simulink model "e5_Quadrotor_stable_nn"  (R2020a)
settings: Solver=FixedStepAuto  StartTime=0.0  StopTime=options.T_train  FixedStep=options.dt  RelTol=1e-6
undefined symbols (not defined in the file or in its folder): options, Quad
libraries: neural x123, simulink x3
(part 1 of 7)
settings Model: Creator=test  LastModifiedBy=kekatos
settings DataIOCC: LimitDataPoints=on  SaveFormat=Array  SignalLoggingSaveFormat=ModelDataLogs  ReturnWorkspaceOutputs=off
settings OptimizationCC: ExpressionDepthLimit=2147483647  LifeSpan=inf
settings DebuggingCC: UnderspecifiedInitializationDetection=Classic  MergeDetectMultiDrivingBlocksExec=none  SolverPrmCheckMsg=warning  FcnCallInpInsideContextMsg=warning  StateNameClashWarn=warning  SFUnexpectedBacktrackingDiag=warning  SFNoUnconditionalDefaultTransitionDiag=warning  SFExecutionAtInitializationDiag=none  ArithmeticOperatorsInVariantConditions=warning
settings HardwareCC: ProdBitPerPointer=32  ProdBitPerSizeT=32  ProdBitPerPtrDiffT=32  ProdLargestAtomicFloat=None  ProdIntDivRoundTo=Undefined  ProdEndianess=Unspecified  ProdWordSize=32  ProdHWDeviceType=32-bit Generic
settings ModelReferenceCC: PropagateSignalLabelsOutOfModel=off
settings SFSimCC: SimUseLocalCustomCode=off  CustomCodeUndefinedFunction=UseInterfaceOnly
settings RTWCC: RTWUseLocalCustomCode=off
settings CodeAppCC: StateflowObjectComments=on
settings GRTTargetCC: TargetLangStandard=C89/C90 (ANSI)  CombineOutputUpdateFcns=off  GRTInterface=on
settings ConfigComp: CovMetricSettings=dw  CovHtmlReporting=on  CovSaveCumulativeToWorkspaceVar=on  CovSaveSingleToWorkspaceVar=on

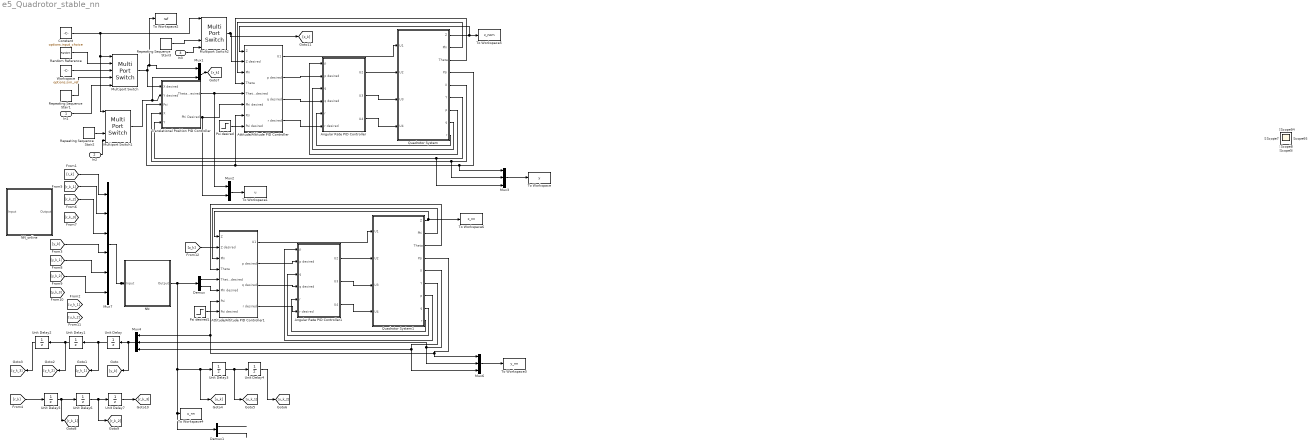
== system e5_Quadrotor_stable_nn ==
  In1 : Inport
  In2 : Inport  Port=2
  In3 : Inport  Port=3
  Angular Rate PID Controller : Subsystem
  Angular Rate PID Controller1 : Subsystem
  Attitude/Altitude PID Controller : Subsystem
  Attitude/Altitude PID Controller1 : Subsystem
  Constant : Constant  Value=options.input_choice
  Demux : Demux  Outputs=2
  Demux1 : Demux  Outputs=2
  Multiport Switch : MultiPortSwitch  Inputs=4
  Multiport Switch1 : MultiPortSwitch  Inputs=4
  Multiport Switch2 : MultiPortSwitch  Inputs=4
  Mux1 : Mux  Inputs=2
  Mux2 : Mux  Inputs=2
  Mux3 : Mux  Inputs=3
  Mux4 : Mux  Inputs=3
  Mux6 : Mux  Inputs=3
  Mux7 : Mux  Inputs=6
  NN : Subsystem
      mask help: Feed-Forward Neural Network
      mask Display: e = 0.06;c1 = [120 150 230]/255;c2 = ([120 150 230]+0)/383;c3 = ([120 150 230]+128)/383;patch([0 1 1 0],[0 0 1 1],c1);patch([0 1 1 1-e 1-e 0+e],[0 0 1 1-e 0+e 0+e],c2);patch([0 0 1 1-e 0+e 0+e],[0 1 1 1-e 1-e 0+e],c3);plot([0 1 1 0 0],[0 0 1 1 0]);fprintf('NNET');port_label('input',1,' Input');port_label('output',1,'Output ');
  NN_online : Subsystem
      mask help: Feed-Forward Neural Network
      mask Display: e = 0.06;c1 = [120 150 230]/255;c2 = ([120 150 230]+0)/383;c3 = ([120 150 230]+128)/383;patch([0 1 1 0],[0 0 1 1],c1);patch([0 1 1 1-e 1-e 0+e],[0 0 1 1-e 0+e 0+e],c2);patch([0 0 1 1-e 0+e 0+e],[0 1 1 1-e 1-e 0+e],c3);plot([0 1 1 0 0],[0 0 1 1 0]);fprintf('NNET');port_label('input',1,' Input');port_label('output',1,'Output ');
  Psi desired : Step  After=0  SampleTime=0
  Psi desired1 : Step  After=0  SampleTime=0
  Quadrotor System : Subsystem
  Quadrotor System1 : Subsystem
  Random Reference : UniformRandomNumber  Minimum=options.ref_min  Maximum=options.ref_max  Seed=randi(2^32,[1 ])  SampleTime=options.ref_Ts
  Repeating Sequence Stair1 : simulink/Sources/Repeating Sequence Stair  OutValues=options.sim_cov  tsamp=options.ref_Ts  OutMin=[]  OutMax=[]  OutDataTypeStr=double  OutputDataTypeScalingMode=double  OutDataType=fixdt(0,8)  ConRadixGroup=Best Precision: Vector-wise  OutScaling=2^-12
  Repeating Sequence Stair2 : simulink/Sources/Repeating Sequence Stair  OutValues=[0.0286;0.0154]  tsamp=options.ref_Ts  OutMin=[]  OutMax=[]  OutDataTypeStr=double  OutputDataTypeScalingMode=double  OutDataType=fixdt(0,8)  ConRadixGroup=Best Precision: Vector-wise  OutScaling=2^-12
  Repeating Sequence Stair3 : simulink/Sources/Repeating Sequence Stair  OutValues=[0.0286;0.0154]  tsamp=options.ref_Ts  OutMin=[]  OutMax=[]  OutDataTypeStr=double  OutputDataTypeScalingMode=double  OutDataType=fixdt(0,8)  ConRadixGroup=Best Precision: Vector-wise  OutScaling=2^-12
  To Workspace : ToWorkspace  VariableName=y  SaveFormat=Structure With Time  SampleTime=0.01
  To Workspace1 : ToWorkspace  VariableName=u  SaveFormat=Structure With Time  SampleTime=0.01
  To Workspace2 : ToWorkspace  VariableName=ref  SaveFormat=Structure With Time  SampleTime=0.01
  To Workspace3 : ToWorkspace  VariableName=y_nn  SaveFormat=Structure With Time  SampleTime=0.01
  To Workspace4 : ToWorkspace  VariableName=u_nn  SaveFormat=Structure With Time  SampleTime=0.01
  To Workspace5 : ToWorkspace  VariableName=z_nom  SaveFormat=Structure With Time  SampleTime=0.01
  To Workspace6 : ToWorkspace  VariableName=z_nn  SaveFormat=Structure With Time  SampleTime=0.01
  Translational Position PID Controller : Subsystem
  Unit Delay{,1..7} (8 alike) : UnitDelay  SampleTime=-1  HasFrameUpgradeWarning=on
  Workspace : Constant  Value=options.sim_ref
  Scope{,1..16} (17 alike) : Scope
  wires:
  Quadrotor System/2(Phi) -> Attitude/Altitude PID Controller/3(Phi)
  Quadrotor System/3(Theta) -> Attitude/Altitude PID Controller/4(Theta)
  Quadrotor System/4(Psi) -> Mux3/1, Translational Position PID Controller/3(Psi), Attitude/Altitude PID Controller/7(Psi)
  Quadrotor System/5(X) -> Mux3/2, Translational Position PID Controller/4(X)
  Quadrotor System/6(Y) -> Mux3/3, Translational Position PID Controller/5(Y)
  Quadrotor System/1(Z) -> To Workspace5/1, Attitude/Altitude PID Controller/1(Z)
  Psi desired/1 -> Attitude/Altitude PID Controller/8(Psi desired)
  Attitude/Altitude PID Controller/1(U1) -> Quadrotor System/1(U1)
  Translational Position PID Controller/1(Theta Desired) -> Mux2/1, Attitude/Altitude PID Controller/5(Theta desired)
  Translational Position PID Controller/2(Phi Desired) -> Attitude/Altitude PID Controller/6(Phi desired), Mux2/2
  Attitude/Altitude PID Controller/2(p desired) -> Angular Rate PID Controller/2(p desired)
  Attitude/Altitude PID Controller/3(q desired) -> Angular Rate PID Controller/4(q desired)
  Attitude/Altitude PID Controller/4(r desired) -> Angular Rate PID Controller/6(r desired)
  Quadrotor System/9(r) -> Angular Rate PID Controller/5(r)
  Quadrotor System/8(q) -> Angular Rate PID Controller/3(q)
  Quadrotor System/7(p) -> Angular Rate PID Controller/1(p)
  Angular Rate PID Controller/3(U4) -> Quadrotor System/4(U4)
  Angular Rate PID Controller/2(U3) -> Quadrotor System/3(U3)
  Angular Rate PID Controller/1(U2) -> Quadrotor System/2(U2)
  Mux2/1 -> To Workspace1/1
  Mux3/1 -> To Workspace/1
  In1/1 -> Multiport Switch/5
  Workspace/1 -> Multiport Switch/3
  Random Reference/1 -> Multiport Switch/2
  Repeating Sequence Stair1/1 -> Multiport Switch/4
  Constant/1 -> Multiport Switch2/1, Multiport Switch1/1, Multiport Switch/1
  Attitude/Altitude PID Controller1/2(p desired) -> Angular Rate PID Controller1/2(p desired)
  Attitude/Altitude PID Controller1/1(U1) -> Quadrotor System1/1(U1)
  Psi desired1/1 -> Attitude/Altitude PID Controller1/8(Psi desired)
  Quadrotor System1/9(r) -> Angular Rate PID Controller1/5(r)
  Quadrotor System1/6(Y) -> Mux4/3, Mux6/3
  Angular Rate PID Controller1/2(U3) -> Quadrotor System1/3(U3)
  Demux/1 -> Attitude/Altitude PID Controller1/5(Theta desired)
  Attitude/Altitude PID Controller1/3(q desired) -> Angular Rate PID Controller1/4(q desired)
  Quadrotor System1/7(p) -> Angular Rate PID Controller1/1(p)
  Quadrotor System1/2(Phi) -> Attitude/Altitude PID Controller1/3(Phi)
  Quadrotor System1/4(Psi) -> Mux6/1, Mux4/1, Attitude/Altitude PID Controller1/7(Psi)
  Demux/2 -> Attitude/Altitude PID Controller1/6(Phi desired)
  Quadrotor System1/3(Theta) -> Attitude/Altitude PID Controller1/4(Theta)
  Angular Rate PID Controller1/1(U2) -> Quadrotor System1/2(U2)
  Quadrotor System1/5(X) -> Mux4/2, Mux6/2
  Angular Rate PID Controller1/3(U4) -> Quadrotor System1/4(U4)
  Quadrotor System1/1(Z) -> Attitude/Altitude PID Controller1/1(Z), To Workspace6/1
  Attitude/Altitude PID Controller1/4(r desired) -> Angular Rate PID Controller1/6(r desired)
  NN/1(Output) -> [u_k], Unit Delay3/1, Demux1/1, To Workspace4/1, Demux/1
  Mux6/1 -> To Workspace3/1
  Quadrotor System1/8(q) -> Angular Rate PID Controller1/3(q)
  Multiport Switch/1 -> Translational Position PID Controller/1(X desired), Mux1/1, To Workspace2/1
  Mux4/1 -> Unit Delay/1, [y_k]
  [r_k] -> Mux7/1
  Mux1/1 -> [r_k]
  Unit Delay/1 -> Unit Delay1/1, [y_k_1]
  Unit Delay1/1 -> Unit Delay2/1, [y_k_2]
  Unit Delay2/1 -> [y_k_3]
  Unit Delay3/1 -> [u_k_1], Unit Delay4/1
  Unit Delay4/1 -> [u_k_2]
  [r_k] -> Unit Delay5/1
  Unit Delay5/1 -> [r_k_1], Unit Delay6/1
  Unit Delay6/1 -> [r_k_2], Unit Delay7/1
  Unit Delay7/1 -> [r_k_3]
  [r_k_1] -> Mux7/2
  [r_k_2] -> Mux7/3
  [y_k] -> Mux7/4
  [y_k_1] -> Mux7/5
  Demux1/1 -> ?
  Demux1/2 -> ?
  Multiport Switch1/1 -> Mux1/2, Translational Position PID Controller/2(Y desired)
  In2/1 -> Multiport Switch1/5
  Repeating Sequence Stair2/1 -> Multiport Switch1/4
  Repeating Sequence Stair3/1 -> Multiport Switch2/4
  In3/1 -> Multiport Switch2/5
  Multiport Switch2/1 -> [z_k], Attitude/Altitude PID Controller/2(Z desired)
  [y_k_2] -> Mux7/6
  [z_k] -> Attitude/Altitude PID Controller1/2(Z desired)
  Mux7/1 -> NN/1(Input)

== system e5_Quadrotor_stable_nn/Angular Rate PID Controller ==
  p : Inport
  p desired : Inport  Port=2
  q : Inport  Port=3
  q desired : Inport  Port=4
  r : Inport  Port=5
  r desired : Inport  Port=6
  p PID : Subsystem
  q PID : Subsystem
  r PID : Subsystem
  U2 : Outport  VectorParamsAs1DForOutWhenUnconnected=off
  U3 : Outport  Port=2  VectorParamsAs1DForOutWhenUnconnected=off
  U4 : Outport  Port=3  VectorParamsAs1DForOutWhenUnconnected=off
  wires:
  p PID/1(U2) -> U2/1
  q PID/1(U3) -> U3/1
  r PID/1(U4) -> U4/1
  p/1 -> p PID/1(p)
  p desired/1 -> p PID/2(p desired)
  q/1 -> q PID/1(q)
  q desired/1 -> q PID/2(q desired)
  r/1 -> r PID/1(r)
  r desired/1 -> r PID/2(r desired)

== system e5_Quadrotor_stable_nn/Angular Rate PID Controller1 ==
  p : Inport
  p desired : Inport  Port=2
  q : Inport  Port=3
  q desired : Inport  Port=4
  r : Inport  Port=5
  r desired : Inport  Port=6
  p PID : Subsystem
  q PID : Subsystem
  r PID : Subsystem
  U2 : Outport  VectorParamsAs1DForOutWhenUnconnected=off
  U3 : Outport  Port=2  VectorParamsAs1DForOutWhenUnconnected=off
  U4 : Outport  Port=3  VectorParamsAs1DForOutWhenUnconnected=off
  wires:
  p PID/1(U2) -> U2/1
  q PID/1(U3) -> U3/1
  r PID/1(U4) -> U4/1
  p/1 -> p PID/1(p)
  p desired/1 -> p PID/2(p desired)
  q/1 -> q PID/1(q)
  q desired/1 -> q PID/2(q desired)
  r/1 -> r PID/1(r)
  r desired/1 -> r PID/2(r desired)

== system e5_Quadrotor_stable_nn/Attitude//Altitude PID Controller ==
  Z : Inport
  Z desired : Inport  Port=2
  Phi : Inport  Port=3
  Theta : Inport  Port=4
  Theta desired : Inport  Port=5
  Phi desired : Inport  Port=6
  Psi : Inport  Port=7
  Psi desired : Inport  Port=8
  Phi PID : Subsystem
  Psi PID : Subsystem
  Theta PID : Subsystem
  Z PID : Subsystem
  U1 : Outport  VectorParamsAs1DForOutWhenUnconnected=off
  p desired : Outport  Port=2  VectorParamsAs1DForOutWhenUnconnected=off
  q desired : Outport  Port=3  VectorParamsAs1DForOutWhenUnconnected=off
  r desired : Outport  Port=4  VectorParamsAs1DForOutWhenUnconnected=off
  wires:
  Z PID/1(U1) -> U1/1
  Z desired/1 -> Z PID/2(Z desired)
  Z/1 -> Z PID/1(Z)
  Phi desired/1 -> Phi PID/2(Phi desired)
  Phi/1 -> Phi PID/1(Phi), Z PID/3(Phi)
  Psi desired/1 -> Psi PID/2(Psi desired)
  Psi/1 -> Psi PID/1(Psi)
  Theta desired/1 -> Theta PID/2(Theta desired)
  Theta/1 -> Theta PID/1(Theta), Z PID/4(Theta)
  Phi PID/1(p desired) -> p desired/1
  Psi PID/1(r desired) -> r desired/1
  Theta PID/1(q desired) -> q desired/1

== system e5_Quadrotor_stable_nn/Attitude//Altitude PID Controller1 ==
  Z : Inport
  Z desired : Inport  Port=2
  Phi : Inport  Port=3
  Theta : Inport  Port=4
  Theta desired : Inport  Port=5
  Phi desired : Inport  Port=6
  Psi : Inport  Port=7
  Psi desired : Inport  Port=8
  Phi PID : Subsystem
  Psi PID : Subsystem
  Theta PID : Subsystem
  Z PID : Subsystem
  U1 : Outport  VectorParamsAs1DForOutWhenUnconnected=off
  p desired : Outport  Port=2  VectorParamsAs1DForOutWhenUnconnected=off
  q desired : Outport  Port=3  VectorParamsAs1DForOutWhenUnconnected=off
  r desired : Outport  Port=4  VectorParamsAs1DForOutWhenUnconnected=off
  wires:
  Z PID/1(U1) -> U1/1
  Z desired/1 -> Z PID/2(Z desired)
  Z/1 -> Z PID/1(Z)
  Phi desired/1 -> Phi PID/2(Phi desired)
  Phi/1 -> Phi PID/1(Phi), Z PID/3(Phi)
  Psi desired/1 -> Psi PID/2(Psi desired)
  Psi/1 -> Psi PID/1(Psi)
  Theta desired/1 -> Theta PID/2(Theta desired)
  Theta/1 -> Theta PID/1(Theta), Z PID/4(Theta)
  Phi PID/1(p desired) -> p desired/1
  Psi PID/1(r desired) -> r desired/1
  Theta PID/1(q desired) -> q desired/1

== system e5_Quadrotor_stable_nn/NN ==
  Input : Inport  PortDimensions=15
      mask Display: e = 0.06;c1 = [120 230 180]/255;c2 = ([120 230 180]+0)/(256+128);c3 = ([120 230 180]+128)/(256+128);patch([0 1 1 0],[0 0 1 1],c1);patch([0 1 1 1-e 1-e 0+e],[0 0 1 1-e 0+e 0+e],c2);patch([0 0 1 1-e 0+e 0+e],[0 1 1 1-e 1-e 0+e],c3);plot([0 1 1 0 0],[0 0 1 1 0]);
  Layer 1 : Subsystem
      mask Display: e = 0.06;c1 = [120 150 230]/255;c2 = ([120 150 230]+0)/383;c3 = ([120 150 230]+128)/383;patch([0 1 1 0],[0 0 1 1],c1);patch([0 1 1 1-e 1-e 0+e],[0 0 1 1-e 0+e 0+e],c2);patch([0 0 1 1-e 0+e 0+e],[0 1 1 1-e 1-e 0+e],c3);plot([0 1 1 0 0],[0 0 1 1 0]);
  Layer 2 : Subsystem
      mask Display: e = 0.06;c1 = [120 150 230]/255;c2 = ([120 150 230]+0)/383;c3 = ([120 150 230]+128)/383;patch([0 1 1 0],[0 0 1 1],c1);patch([0 1 1 1-e 1-e 0+e],[0 0 1 1-e 0+e 0+e],c2);patch([0 0 1 1-e 0+e 0+e],[0 1 1 1-e 1-e 0+e],c3);plot([0 1 1 0 0],[0 0 1 1 0]);
  Process Input 1 : Subsystem
      mask Display: e = 0.06;c1 = [120 150 230]/255;c2 = ([120 150 230]+0)/383;c3 = ([120 150 230]+128)/383;patch([0 1 1 0],[0 0 1 1],c1);patch([0 1 1 1-e 1-e 0+e],[0 0 1 1-e 0+e 0+e],c2);patch([0 0 1 1-e 0+e 0+e],[0 1 1 1-e 1-e 0+e],c3);plot([0 1 1 0 0],[0 0 1 1 0]);
  Process Output 1 : Subsystem
      mask Display: e = 0.06;c1 = [120 150 230]/255;c2 = ([120 150 230]+0)/383;c3 = ([120 150 230]+128)/383;patch([0 1 1 0],[0 0 1 1],c1);patch([0 1 1 1-e 1-e 0+e],[0 0 1 1-e 0+e 0+e],c2);patch([0 0 1 1-e 0+e 0+e],[0 1 1 1-e 1-e 0+e],c3);plot([0 1 1 0 0],[0 0 1 1 0]);
  Output : Outport  InitialOutput=[0;0]
      mask Display: e = 0.06;c1 = [120 230 180]/255;c2 = ([120 230 180]+0)/(256+128);c3 = ([120 230 180]+128)/(256+128);patch([0 1 1 0],[0 0 1 1],c1);patch([0 1 1 1-e 1-e 0+e],[0 0 1 1-e 0+e 0+e],c2);patch([0 0 1 1-e 0+e 0+e],[0 1 1 1-e 1-e 0+e],c3);plot([0 1 1 0 0],[0 0 1 1 0]);
  wires:
  Input/1 -> Process Input 1/1(x)
  Process Output 1/1(y) -> Output/1
  Process Input 1/1(p) -> Layer 1/1("p{1}")
  Layer 1/1("a{1}") -> [feedback1]
  [feedback1] -> Layer 2/1("a{1} ")
  Layer 2/1("a{2}") -> Process Output 1/1(a)

== system e5_Quadrotor_stable_nn/NN_online ==
  Input : Inport  PortDimensions=20
      mask Display: e = 0.06;c1 = [120 230 180]/255;c2 = ([120 230 180]+0)/(256+128);c3 = ([120 230 180]+128)/(256+128);patch([0 1 1 0],[0 0 1 1],c1);patch([0 1 1 1-e 1-e 0+e],[0 0 1 1-e 0+e 0+e],c2);patch([0 0 1 1-e 0+e 0+e],[0 1 1 1-e 1-e 0+e],c3);plot([0 1 1 0 0],[0 0 1 1 0]);
  Layer 1 : Subsystem
      mask Display: e = 0.06;c1 = [120 150 230]/255;c2 = ([120 150 230]+0)/383;c3 = ([120 150 230]+128)/383;patch([0 1 1 0],[0 0 1 1],c1);patch([0 1 1 1-e 1-e 0+e],[0 0 1 1-e 0+e 0+e],c2);patch([0 0 1 1-e 0+e 0+e],[0 1 1 1-e 1-e 0+e],c3);plot([0 1 1 0 0],[0 0 1 1 0]);
  Layer 2 : Subsystem
      mask Display: e = 0.06;c1 = [120 150 230]/255;c2 = ([120 150 230]+0)/383;c3 = ([120 150 230]+128)/383;patch([0 1 1 0],[0 0 1 1],c1);patch([0 1 1 1-e 1-e 0+e],[0 0 1 1-e 0+e 0+e],c2);patch([0 0 1 1-e 0+e 0+e],[0 1 1 1-e 1-e 0+e],c3);plot([0 1 1 0 0],[0 0 1 1 0]);
  Layer 3 : Subsystem
      mask Display: e = 0.06;c1 = [120 150 230]/255;c2 = ([120 150 230]+0)/383;c3 = ([120 150 230]+128)/383;patch([0 1 1 0],[0 0 1 1],c1);patch([0 1 1 1-e 1-e 0+e],[0 0 1 1-e 0+e 0+e],c2);patch([0 0 1 1-e 0+e 0+e],[0 1 1 1-e 1-e 0+e],c3);plot([0 1 1 0 0],[0 0 1 1 0]);
  Process Input 1 : Subsystem
      mask Display: e = 0.06;c1 = [120 150 230]/255;c2 = ([120 150 230]+0)/383;c3 = ([120 150 230]+128)/383;patch([0 1 1 0],[0 0 1 1],c1);patch([0 1 1 1-e 1-e 0+e],[0 0 1 1-e 0+e 0+e],c2);patch([0 0 1 1-e 0+e 0+e],[0 1 1 1-e 1-e 0+e],c3);plot([0 1 1 0 0],[0 0 1 1 0]);
  Process Output 1 : Subsystem
      mask Display: e = 0.06;c1 = [120 150 230]/255;c2 = ([120 150 230]+0)/383;c3 = ([120 150 230]+128)/383;patch([0 1 1 0],[0 0 1 1],c1);patch([0 1 1 1-e 1-e 0+e],[0 0 1 1-e 0+e 0+e],c2);patch([0 0 1 1-e 0+e 0+e],[0 1 1 1-e 1-e 0+e],c3);plot([0 1 1 0 0],[0 0 1 1 0]);
  Output : Outport  InitialOutput=[0;0]
      mask Display: e = 0.06;c1 = [120 230 180]/255;c2 = ([120 230 180]+0)/(256+128);c3 = ([120 230 180]+128)/(256+128);patch([0 1 1 0],[0 0 1 1],c1);patch([0 1 1 1-e 1-e 0+e],[0 0 1 1-e 0+e 0+e],c2);patch([0 0 1 1-e 0+e 0+e],[0 1 1 1-e 1-e 0+e],c3);plot([0 1 1 0 0],[0 0 1 1 0]);
  wires:
  Input/1 -> Process Input 1/1(x)
  Process Output 1/1(y) -> Output/1
  Process Input 1/1(p) -> Layer 1/1("p{1}")
  Layer 1/1("a{1}") -> [feedback1]
  [feedback1] -> Layer 2/1("a{1} ")
  Layer 2/1("a{2}") -> [feedback2]
  [feedback2] -> Layer 3/1("a{2} ")
  Layer 3/1("a{3}") -> Process Output 1/1(a)

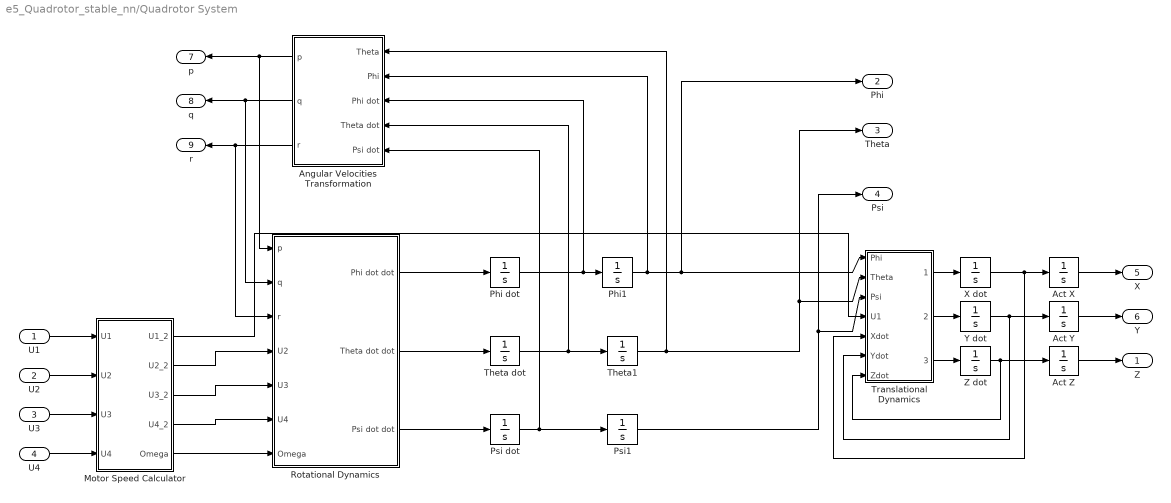
== system e5_Quadrotor_stable_nn/Quadrotor System ==
  U1 : Inport
  U2 : Inport  Port=2
  U3 : Inport  Port=3
  U4 : Inport  Port=4
  Act X : Integrator
  Act Y : Integrator
  Act Z : Integrator
  Angular Velocities Transformation : Subsystem
  Motor Speed Calculator : Subsystem
  Phi dot : Integrator
  Phi1 : Integrator  ZeroCross=off
  Psi dot : Integrator  ZeroCross=off
  Psi1 : Integrator  ZeroCross=off
  Rotational Dynamics : Subsystem
  Theta dot : Integrator  ZeroCross=off
  Theta1 : Integrator  ZeroCross=off
  Translational Dynamics : Subsystem
  X dot : Integrator
  Y dot : Integrator
  Z dot : Integrator
  Z : Outport  VectorParamsAs1DForOutWhenUnconnected=off
  Phi : Outport  Port=2  VectorParamsAs1DForOutWhenUnconnected=off
  Theta : Outport  Port=3  VectorParamsAs1DForOutWhenUnconnected=off
  Psi : Outport  Port=4  VectorParamsAs1DForOutWhenUnconnected=off
  X : Outport  Port=5  VectorParamsAs1DForOutWhenUnconnected=off
  Y : Outport  Port=6  VectorParamsAs1DForOutWhenUnconnected=off
  p : Outport  Port=7  VectorParamsAs1DForOutWhenUnconnected=off
  q : Outport  Port=8  VectorParamsAs1DForOutWhenUnconnected=off
  r : Outport  Port=9  VectorParamsAs1DForOutWhenUnconnected=off
  wires:
  Rotational Dynamics/2(Theta dot dot) -> Theta dot/1
  Motor Speed Calculator/5(Omega) -> Rotational Dynamics/7(Omega)
  Phi1/1 -> Translational Dynamics/1(Phi), Phi/1, Angular Velocities Transformation/2(Phi)
  Theta1/1 -> Translational Dynamics/2(Theta), Theta/1, Angular Velocities Transformation/1(Theta)
  Psi1/1 -> Translational Dynamics/3(Psi), Psi/1
  Translational Dynamics/1(x dotdot) -> X dot/1
  X dot/1 -> Act X/1, Translational Dynamics/5(Xdot)
  Y dot/1 -> Act Y/1, Translational Dynamics/6(Ydot)
  Translational Dynamics/2(y dotdot) -> Y dot/1
  Z dot/1 -> Translational Dynamics/7(Zdot), Act Z/1
  Translational Dynamics/3(z dotdot) -> Z dot/1
  Act X/1 -> X/1
  Act Y/1 -> Y/1
  Act Z/1 -> Z/1
  Psi dot/1 -> Psi1/1, Angular Velocities Transformation/5(Psi dot)
  Theta dot/1 -> Theta1/1, Angular Velocities Transformation/4(Theta dot)
  Phi dot/1 -> Phi1/1, Angular Velocities Transformation/3(Phi dot)
  Rotational Dynamics/3(Psi dot dot) -> Psi dot/1
  Rotational Dynamics/1(Phi dot dot) -> Phi dot/1
  U4/1 -> Motor Speed Calculator/4(U4)
  U2/1 -> Motor Speed Calculator/2(U2)
  U3/1 -> Motor Speed Calculator/3(U3)
  Motor Speed Calculator/2(U2_2) -> Rotational Dynamics/4(U2)
  Motor Speed Calculator/3(U3_2) -> Rotational Dynamics/5(U3)
  Motor Speed Calculator/1(U1_2) -> Translational Dynamics/4(U1)
  Motor Speed Calculator/4(U4_2) -> Rotational Dynamics/6(U4)
  Angular Velocities Transformation/1(p) -> Rotational Dynamics/1(p), p/1
  Angular Velocities Transformation/2(q) -> Rotational Dynamics/2(q), q/1
  Angular Velocities Transformation/3(r) -> Rotational Dynamics/3(r), r/1
  U1/1 -> Motor Speed Calculator/1(U1)

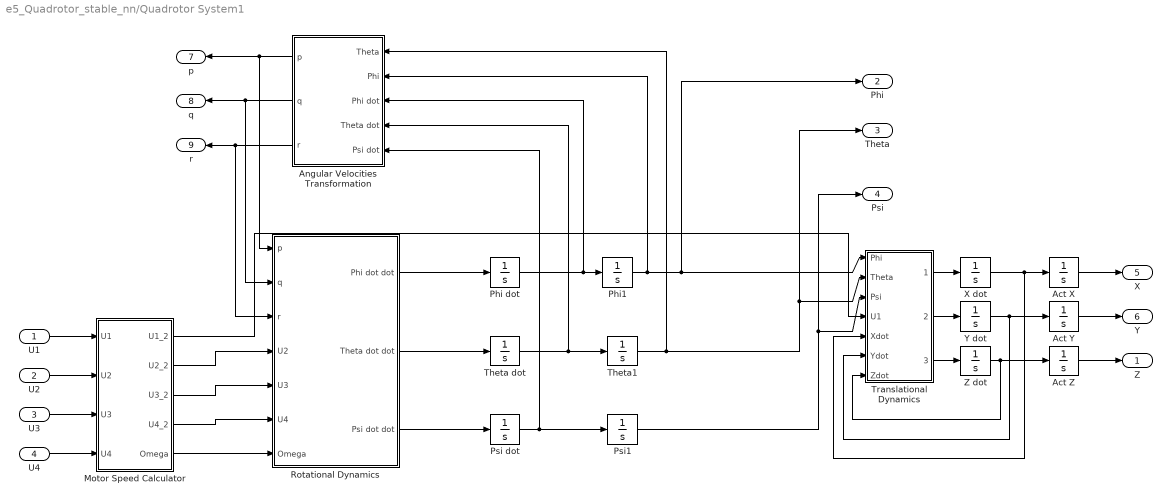
== system e5_Quadrotor_stable_nn/Quadrotor System1 ==
  U1 : Inport
  U2 : Inport  Port=2
  U3 : Inport  Port=3
  U4 : Inport  Port=4
  Act X : Integrator
  Act Y : Integrator
  Act Z : Integrator
  Angular Velocities Transformation : Subsystem
  Motor Speed Calculator : Subsystem
  Phi dot : Integrator
  Phi1 : Integrator  ZeroCross=off
  Psi dot : Integrator  ZeroCross=off
  Psi1 : Integrator  ZeroCross=off
  Rotational Dynamics : Subsystem
  Theta dot : Integrator  ZeroCross=off
  Theta1 : Integrator  ZeroCross=off
  Translational Dynamics : Subsystem
  X dot : Integrator
  Y dot : Integrator
  Z dot : Integrator
  Z : Outport  VectorParamsAs1DForOutWhenUnconnected=off
  Phi : Outport  Port=2  VectorParamsAs1DForOutWhenUnconnected=off
  Theta : Outport  Port=3  VectorParamsAs1DForOutWhenUnconnected=off
  Psi : Outport  Port=4  VectorParamsAs1DForOutWhenUnconnected=off
  X : Outport  Port=5  VectorParamsAs1DForOutWhenUnconnected=off
  Y : Outport  Port=6  VectorParamsAs1DForOutWhenUnconnected=off
  p : Outport  Port=7  VectorParamsAs1DForOutWhenUnconnected=off
  q : Outport  Port=8  VectorParamsAs1DForOutWhenUnconnected=off
  r : Outport  Port=9  VectorParamsAs1DForOutWhenUnconnected=off
  wires:
  Rotational Dynamics/2(Theta dot dot) -> Theta dot/1
  Motor Speed Calculator/5(Omega) -> Rotational Dynamics/7(Omega)
  Phi1/1 -> Translational Dynamics/1(Phi), Phi/1, Angular Velocities Transformation/2(Phi)
  Theta1/1 -> Translational Dynamics/2(Theta), Theta/1, Angular Velocities Transformation/1(Theta)
  Psi1/1 -> Translational Dynamics/3(Psi), Psi/1
  Translational Dynamics/1(x dotdot) -> X dot/1
  X dot/1 -> Act X/1, Translational Dynamics/5(Xdot)
  Y dot/1 -> Act Y/1, Translational Dynamics/6(Ydot)
  Translational Dynamics/2(y dotdot) -> Y dot/1
  Z dot/1 -> Translational Dynamics/7(Zdot), Act Z/1
  Translational Dynamics/3(z dotdot) -> Z dot/1
  Act X/1 -> X/1
  Act Y/1 -> Y/1
  Act Z/1 -> Z/1
  Psi dot/1 -> Psi1/1, Angular Velocities Transformation/5(Psi dot)
  Theta dot/1 -> Theta1/1, Angular Velocities Transformation/4(Theta dot)
  Phi dot/1 -> Phi1/1, Angular Velocities Transformation/3(Phi dot)
  Rotational Dynamics/3(Psi dot dot) -> Psi dot/1
  Rotational Dynamics/1(Phi dot dot) -> Phi dot/1
  U4/1 -> Motor Speed Calculator/4(U4)
  U2/1 -> Motor Speed Calculator/2(U2)
  U3/1 -> Motor Speed Calculator/3(U3)
  Motor Speed Calculator/2(U2_2) -> Rotational Dynamics/4(U2)
  Motor Speed Calculator/3(U3_2) -> Rotational Dynamics/5(U3)
  Motor Speed Calculator/1(U1_2) -> Translational Dynamics/4(U1)
  Motor Speed Calculator/4(U4_2) -> Rotational Dynamics/6(U4)
  Angular Velocities Transformation/1(p) -> Rotational Dynamics/1(p), p/1
  Angular Velocities Transformation/2(q) -> Rotational Dynamics/2(q), q/1
  Angular Velocities Transformation/3(r) -> Rotational Dynamics/3(r), r/1
  U1/1 -> Motor Speed Calculator/1(U1)

== system e5_Quadrotor_stable_nn/Translational Position PID Controller ==
  X desired : Inport
  Y desired : Inport  Port=2
  Psi : Inport  Port=3
  X : Inport  Port=4
  Y : Inport  Port=5
  Desired Position GF to BF : Subsystem
  Position GF to BF : Subsystem
  X PID : Subsystem
  Y PID : Subsystem
  Theta Desired : Outport  VectorParamsAs1DForOutWhenUnconnected=off
  Phi Desired : Outport  Port=2  VectorParamsAs1DForOutWhenUnconnected=off
  wires:
  X PID/1(Theta Desired) -> Theta Desired/1
  Y PID/1(Phi Desired) -> Phi Desired/1
  X desired/1 -> Desired Position GF to BF/1(X GF)
  Y desired/1 -> Desired Position GF to BF/2(Y GF)
  Desired Position GF to BF/1("X Bf ") -> X PID/1(X desired)
  Desired Position GF to BF/2(Y Bf) -> Y PID/1(Y desired)
  X/1 -> Position GF to BF/1(X GF)
  Y/1 -> Position GF to BF/2(Y GF)
  Position GF to BF/1("X Bf ") -> X PID/2(X)
  Position GF to BF/2(Y Bf) -> Y PID/2(Y)
  Psi/1 -> Desired Position GF to BF/3(Psi), Position GF to BF/3(Psi)

== system e5_Quadrotor_stable_nn/Angular Rate PID Controller/p PID ==
  p : Inport
  p desired : Inport  Port=2
  Derivative : Derivative
  Integrator : Integrator
  Kd : Gain  Gain=Quad.p_KD
  Ki : Gain  Gain=Quad.p_KI
  Kp : Gain  Gain=Quad.p_KP
  Psi Error : Sum  Inputs=+-
  Saturation1 : Saturate  UpperLimit=Quad.U2_max  LowerLimit=Quad.U2_min
  Sum : Sum  Inputs=+++
  U2 : Outport  VectorParamsAs1DForOutWhenUnconnected=off
  wires:
  p/1 -> Psi Error/2, Derivative/1
  p desired/1 -> Psi Error/1
  Derivative/1 -> Kd/1
  Kp/1 -> Sum/1
  Sum/1 -> U2/1
  Psi Error/1 -> Integrator/1, Kp/1
  Integrator/1 -> Ki/1
  Kd/1 -> Sum/3
  Ki/1 -> Saturation1/1
  Saturation1/1 -> Sum/2

== system e5_Quadrotor_stable_nn/Angular Rate PID Controller/q PID ==
  q : Inport
  q desired : Inport  Port=2
  Derivative : Derivative
  Integrator : Integrator
  Kd : Gain  Gain=Quad.q_KD
  Ki : Gain  Gain=Quad.q_KI
  Kp : Gain  Gain=Quad.q_KP
  Saturation1 : Saturate  UpperLimit=Quad.U3_max  LowerLimit=Quad.U3_min
  Scope : Scope
  Sum : Sum  Inputs=+++
  q Error : Sum  Inputs=+-
  U3 : Outport  VectorParamsAs1DForOutWhenUnconnected=off
  wires:
  q/1 -> q Error/2, Derivative/1
  q desired/1 -> q Error/1
  Derivative/1 -> Kd/1
  Kp/1 -> Sum/1
  Sum/1 -> U3/1
  q Error/1 -> Integrator/1, Kp/1, Scope/1
  Integrator/1 -> Ki/1
  Kd/1 -> Sum/3
  Ki/1 -> Saturation1/1
  Saturation1/1 -> Sum/2

== system e5_Quadrotor_stable_nn/Angular Rate PID Controller/r PID ==
  r : Inport
  r desired : Inport  Port=2
  Derivative : Derivative
  Integrator : Integrator
  Kd : Gain  Gain=Quad.r_KD
  Ki : Gain  Gain=Quad.r_KI
  Kp : Gain  Gain=Quad.r_KP
  Psi Error : Sum  Inputs=+-
  Sum : Sum  Inputs=+++
  U4 : Outport  VectorParamsAs1DForOutWhenUnconnected=off
  wires:
  r/1 -> Psi Error/2, Derivative/1
  r desired/1 -> Psi Error/1
  Derivative/1 -> Kd/1
  Kp/1 -> Sum/1
  Sum/1 -> U4/1
  Psi Error/1 -> Integrator/1, Kp/1
  Integrator/1 -> Ki/1
  Kd/1 -> Sum/3

== system e5_Quadrotor_stable_nn/Angular Rate PID Controller1/p PID ==
  p : Inport
  p desired : Inport  Port=2
  Derivative : Derivative
  Integrator : Integrator
  Kd : Gain  Gain=Quad.p_KD
  Ki : Gain  Gain=Quad.p_KI
  Kp : Gain  Gain=Quad.p_KP
  Psi Error : Sum  Inputs=+-
  Saturation1 : Saturate  UpperLimit=Quad.U2_max  LowerLimit=Quad.U2_min
  Sum : Sum  Inputs=+++
  U2 : Outport  VectorParamsAs1DForOutWhenUnconnected=off
  wires:
  p/1 -> Psi Error/2, Derivative/1
  p desired/1 -> Psi Error/1
  Derivative/1 -> Kd/1
  Kp/1 -> Sum/1
  Sum/1 -> U2/1
  Psi Error/1 -> Integrator/1, Kp/1
  Integrator/1 -> Ki/1
  Kd/1 -> Sum/3
  Ki/1 -> Saturation1/1
  Saturation1/1 -> Sum/2

== system e5_Quadrotor_stable_nn/Angular Rate PID Controller1/q PID ==
  q : Inport
  q desired : Inport  Port=2
  Derivative : Derivative
  Integrator : Integrator
  Kd : Gain  Gain=Quad.q_KD
  Ki : Gain  Gain=Quad.q_KI
  Kp : Gain  Gain=Quad.q_KP
  Saturation1 : Saturate  UpperLimit=Quad.U3_max  LowerLimit=Quad.U3_min
  Scope : Scope
  Sum : Sum  Inputs=+++
  q Error : Sum  Inputs=+-
  U3 : Outport  VectorParamsAs1DForOutWhenUnconnected=off
  wires:
  q/1 -> q Error/2, Derivative/1
  q desired/1 -> q Error/1
  Derivative/1 -> Kd/1
  Kp/1 -> Sum/1
  Sum/1 -> U3/1
  q Error/1 -> Integrator/1, Kp/1, Scope/1
  Integrator/1 -> Ki/1
  Kd/1 -> Sum/3
  Ki/1 -> Saturation1/1
  Saturation1/1 -> Sum/2

== system e5_Quadrotor_stable_nn/Angular Rate PID Controller1/r PID ==
  r : Inport
  r desired : Inport  Port=2
  Derivative : Derivative
  Integrator : Integrator
  Kd : Gain  Gain=Quad.r_KD
  Ki : Gain  Gain=Quad.r_KI
  Kp : Gain  Gain=Quad.r_KP
  Psi Error : Sum  Inputs=+-
  Sum : Sum  Inputs=+++
  U4 : Outport  VectorParamsAs1DForOutWhenUnconnected=off
  wires:
  r/1 -> Psi Error/2, Derivative/1
  r desired/1 -> Psi Error/1
  Derivative/1 -> Kd/1
  Kp/1 -> Sum/1
  Sum/1 -> U4/1
  Psi Error/1 -> Integrator/1, Kp/1
  Integrator/1 -> Ki/1
  Kd/1 -> Sum/3

== system e5_Quadrotor_stable_nn/Attitude//Altitude PID Controller/Phi PID ==
  Phi : Inport
  Phi desired : Inport  Port=2
  Derivative : Derivative
  Integrator : Integrator
  Kd : Gain  Gain=Quad.phi_KD
  Ki : Gain  Gain=Quad.phi_KI
  Kp : Gain  Gain=Quad.phi_KP
  Psi Error : Sum  Inputs=+-
  Sum : Sum  Inputs=+++
  p desired : Outport  VectorParamsAs1DForOutWhenUnconnected=off
  wires:
  Phi/1 -> Psi Error/2, Derivative/1
  Phi desired/1 -> Psi Error/1
  Derivative/1 -> Kd/1
  Kp/1 -> Sum/1
  Sum/1 -> p desired/1
  Psi Error/1 -> Integrator/1, Kp/1
  Integrator/1 -> Ki/1
  Kd/1 -> Sum/3
  Ki/1 -> Sum/2

== system e5_Quadrotor_stable_nn/Attitude//Altitude PID Controller/Psi PID ==
  Psi : Inport
  Psi desired : Inport  Port=2
  Derivative : Derivative
  Integrator : Integrator
  Kd : Gain  Gain=Quad.psi_KD
  Ki : Gain  Gain=Quad.psi_KI
  Kp : Gain  Gain=Quad.psi_KP
  Psi Error : Sum  Inputs=+-
  Sum : Sum  Inputs=+++
  r desired : Outport  VectorParamsAs1DForOutWhenUnconnected=off
  wires:
  Psi/1 -> Psi Error/2, Derivative/1
  Psi desired/1 -> Psi Error/1
  Derivative/1 -> Kd/1
  Kp/1 -> Sum/1
  Sum/1 -> r desired/1
  Psi Error/1 -> Integrator/1, Kp/1
  Integrator/1 -> Ki/1
  Kd/1 -> Sum/3
  Ki/1 -> Sum/2

== system e5_Quadrotor_stable_nn/Attitude//Altitude PID Controller/Theta PID ==
  Theta : Inport
  Theta desired : Inport  Port=2
  Derivative : Derivative
  Integrator : Integrator
  Kd : Gain  Gain=Quad.theta_KD
  Ki : Gain  Gain=Quad.theta_KI
  Kp : Gain  Gain=Quad.theta_KP
  Scope : Scope
  Sum : Sum  Inputs=+++
  Theta Error : Sum  Inputs=+-
  q desired : Outport  VectorParamsAs1DForOutWhenUnconnected=off
  wires:
  Theta/1 -> Theta Error/2, Derivative/1
  Theta desired/1 -> Theta Error/1
  Derivative/1 -> Kd/1
  Kp/1 -> Sum/1
  Sum/1 -> q desired/1
  Theta Error/1 -> Integrator/1, Kp/1, Scope/1
  Integrator/1 -> Ki/1
  Kd/1 -> Sum/3
  Ki/1 -> Sum/2

== system e5_Quadrotor_stable_nn/Attitude//Altitude PID Controller/Z PID ==
  Z : Inport
  Z desired : Inport  Port=2
  Phi : Inport  Port=3
  Theta : Inport  Port=4
  Derivative : Derivative
  Divide : Product  Inputs=*/
  Integrator : Integrator
  Kd : Gain  Gain=Quad.Z_KD
  Ki : Gain  Gain=Quad.Z_KI
  Kp : Gain  Gain=Quad.Z_KP
  Product : Product  RndMeth=Zero
  Sum : Sum  Inputs=---+
  cos Phi : Trigonometry  Operator=cos
  cos Theta : Trigonometry  Operator=cos
  ez : Sum  Inputs=+-
  mg : Constant  Value=Quad.m*Quad.g
  U1 : Outport  VectorParamsAs1DForOutWhenUnconnected=off
  wires:
  Z desired/1 -> ez/1
  cos Phi/1 -> Product/1
  cos Theta/1 -> Product/2
  Product/1 -> Divide/2
  Phi/1 -> cos Phi/1
  Theta/1 -> cos Theta/1
  Z/1 -> ez/2, Derivative/1
  Derivative/1 -> Kd/1
  Kp/1 -> Sum/1
  Integrator/1 -> Ki/1
  ez/1 -> Integrator/1, Kp/1
  Sum/1 -> Divide/1
  Divide/1 -> U1/1
  mg/1 -> Sum/4
  Kd/1 -> Sum/3
  Ki/1 -> Sum/2

== system e5_Quadrotor_stable_nn/Attitude//Altitude PID Controller1/Phi PID ==
  Phi : Inport
  Phi desired : Inport  Port=2
  Derivative : Derivative
  Integrator : Integrator
  Kd : Gain  Gain=Quad.phi_KD
  Ki : Gain  Gain=Quad.phi_KI
  Kp : Gain  Gain=Quad.phi_KP
  Psi Error : Sum  Inputs=+-
  Sum : Sum  Inputs=+++
  p desired : Outport  VectorParamsAs1DForOutWhenUnconnected=off
  wires:
  Phi/1 -> Psi Error/2, Derivative/1
  Phi desired/1 -> Psi Error/1
  Derivative/1 -> Kd/1
  Kp/1 -> Sum/1
  Sum/1 -> p desired/1
  Psi Error/1 -> Integrator/1, Kp/1
  Integrator/1 -> Ki/1
  Kd/1 -> Sum/3
  Ki/1 -> Sum/2

== system e5_Quadrotor_stable_nn/Attitude//Altitude PID Controller1/Psi PID ==
  Psi : Inport
  Psi desired : Inport  Port=2
  Derivative : Derivative
  Integrator : Integrator
  Kd : Gain  Gain=Quad.psi_KD
  Ki : Gain  Gain=Quad.psi_KI
  Kp : Gain  Gain=Quad.psi_KP
  Psi Error : Sum  Inputs=+-
  Sum : Sum  Inputs=+++
  r desired : Outport  VectorParamsAs1DForOutWhenUnconnected=off
  wires:
  Psi/1 -> Psi Error/2, Derivative/1
  Psi desired/1 -> Psi Error/1
  Derivative/1 -> Kd/1
  Kp/1 -> Sum/1
  Sum/1 -> r desired/1
  Psi Error/1 -> Integrator/1, Kp/1
  Integrator/1 -> Ki/1
  Kd/1 -> Sum/3
  Ki/1 -> Sum/2

== system e5_Quadrotor_stable_nn/Attitude//Altitude PID Controller1/Theta PID ==
  Theta : Inport
  Theta desired : Inport  Port=2
  Derivative : Derivative
  Integrator : Integrator
  Kd : Gain  Gain=Quad.theta_KD
  Ki : Gain  Gain=Quad.theta_KI
  Kp : Gain  Gain=Quad.theta_KP
  Scope : Scope
  Sum : Sum  Inputs=+++
  Theta Error : Sum  Inputs=+-
  q desired : Outport  VectorParamsAs1DForOutWhenUnconnected=off
  wires:
  Theta/1 -> Theta Error/2, Derivative/1
  Theta desired/1 -> Theta Error/1
  Derivative/1 -> Kd/1
  Kp/1 -> Sum/1
  Sum/1 -> q desired/1
  Theta Error/1 -> Integrator/1, Kp/1, Scope/1
  Integrator/1 -> Ki/1
  Kd/1 -> Sum/3
  Ki/1 -> Sum/2

== system e5_Quadrotor_stable_nn/Attitude//Altitude PID Controller1/Z PID ==
  Z : Inport
  Z desired : Inport  Port=2
  Phi : Inport  Port=3
  Theta : Inport  Port=4
  Derivative : Derivative
  Divide : Product  Inputs=*/
  Integrator : Integrator
  Kd : Gain  Gain=Quad.Z_KD
  Ki : Gain  Gain=Quad.Z_KI
  Kp : Gain  Gain=Quad.Z_KP
  Product : Product  RndMeth=Zero
  Sum : Sum  Inputs=---+
  cos Phi : Trigonometry  Operator=cos
  cos Theta : Trigonometry  Operator=cos
  ez : Sum  Inputs=+-
  mg : Constant  Value=Quad.m*Quad.g
  U1 : Outport  VectorParamsAs1DForOutWhenUnconnected=off
  wires:
  Z desired/1 -> ez/1
  cos Phi/1 -> Product/1
  cos Theta/1 -> Product/2
  Product/1 -> Divide/2
  Phi/1 -> cos Phi/1
  Theta/1 -> cos Theta/1
  Z/1 -> ez/2, Derivative/1
  Derivative/1 -> Kd/1
  Kp/1 -> Sum/1
  Integrator/1 -> Ki/1
  ez/1 -> Integrator/1, Kp/1
  Sum/1 -> Divide/1
  Divide/1 -> U1/1
  mg/1 -> Sum/4
  Kd/1 -> Sum/3
  Ki/1 -> Sum/2

== system e5_Quadrotor_stable_nn/NN/Layer 1 ==
  "p{1}" : Inport  PortDimensions=15
      mask Display: e = 0.06;c1 = [120 230 180]/255;c2 = ([120 230 180]+0)/(256+128);c3 = ([120 230 180]+128)/(256+128);patch([0 1 1 0],[0 0 1 1],c1);patch([0 1 1 1-e 1-e 0+e],[0 0 1 1-e 0+e 0+e],c2);patch([0 0 1 1-e 0+e 0+e],[0 1 1 1-e 1-e 0+e],c3);plot([0 1 1 0 0],[0 0 1 1 0]);
  Delays 1 : Subsystem
      mask Display: e = 0.06;c1 = [120 150 230]/255;c2 = ([120 150 230]+0)/383;c3 = ([120 150 230]+128)/383;patch([0 1 1 0],[0 0 1 1],c1);patch([0 1 1 1-e 1-e 0+e],[0 0 1 1-e 0+e 0+e],c2);patch([0 0 1 1-e 0+e 0+e],[0 1 1 1-e 1-e 0+e],c3);plot([0 1 1 0 0],[0 0 1 1 0]);disp('0');
  "IW{1,1}" : Subsystem
      mask Display: e = 0.06;c1 = [120 150 230]/255;c2 = ([120 150 230]+0)/383;c3 = ([120 150 230]+128)/383;patch([0 1 1 0],[0 0 1 1],c1);patch([0 1 1 1-e 1-e 0+e],[0 0 1 1-e 0+e 0+e],c2);patch([0 0 1 1-e 0+e 0+e],[0 1 1 1-e 1-e 0+e],c3);plot([0 1 1 0 0],[0 0 1 1 0]);disp('W');
  "b{1}" : Constant  Value=[-1.84537637140731280993577456683851778507232666015625;-1.7532825244992047419856362466816790401935577392578125;1.71407838156578673505237020435743033885955810546875;-1.6342052333083547654979383878526277840137481689453125;-1.5438537489742396591196893496089614927768707275390625;1.4283080018807214894849266784149222075939178466796875;-1.404821018307291780047307838685810565948486328125;1.287885767879537457503147379611618816852569580078125;1.25502611674529962471069666207768023014068603515625;1.0972360429977421336644738403265364468097686767578125;1.131430962279293073180497231078334152698516845703125;-0.9955530066140656497708505412447266280651092529296875;-0.89412837469389450095746951774344779551029205322265625;0.85010871782267416474354604360996745526790618896484375;-0.80545016544390790613761055283248424530029296875;-0.70922638754411959638446205644868314266204833984375;-0.63105719893839429257553774732514284551143646240234375;-0.569988447775239048809226005687378346920013427734375;0.477593047053590902262243389486684463918209075927734375;0.403175590821758189630230617694905959069728851318359375;0.358673720801043760531001680647023022174835205078125;-0.2482304075266782150688271713079302571713924407958984375;0.15068110824116487389545682162861339747905731201171875;-0.1602803495511306020038233555169426836073398590087890625;-0.0987868360797714839538485875891637988388538360595703125;0.04171171965434290751506551941929501481354236602783203125;0.0939112815207025775077198659346322529017925262451171875;-0.177186006071735346889539641779265366494655609130859375;0.2396368639811528866712109220316051505506038665771484375;0.342981184701568242445546275121159851551055908203125;0.416928111920932209510937127561192028224468231201171875;-0.495950560740119616998100582350161857903003692626953125;-0.590456977511941705216713671688921749591827392578125;-0.6649151320152437705246484256349503993988037109375;-0.608626845880423150703109058667905628681182861328125;0.79801769557657376008563687719288282096385955810546875;0.89966865010810692648846043084631673991680145263671875;0.9564815597009614922541231862851418554782867431640625;-1.04442351552266732284124373109079897403717041015625;-1.0713399950107189706471899626194499433040618896484375;-1.191236975152814903111675448599271476268768310546875;-1.1699716443134151599991810144274495542049407958984375;-1.29708105375885995869111866340972483158111572265625;1.3771740284091971151525513050728477537631988525390625;1.3780962923269959308214538395986892282962799072265625;1.53107763486454206969256119919009506702423095703125;-1.625607738312811800795998351532034575939178466796875;-1.698033535260649262710330731351859867572784423828125;-1.740593156442128641714361947379074990749359130859375;-1.7825772239617221348595421659410931169986724853515625]
      mask Display: e = 0.06;c1 = [120 150 230]/255;c2 = ([120 150 230]+0)/383;c3 = ([120 150 230]+128)/383;patch([0 1 1 0],[0 0 1 1],c1);patch([0 1 1 1-e 1-e 0+e],[0 0 1 1-e 0+e 0+e],c2);patch([0 0 1 1-e 0+e 0+e],[0 1 1 1-e 1-e 0+e],c3);plot([0 1 1 0 0],[0 0 1 1 0]);disp('b');
  netsum : Sum  Inputs=2  InputSameDT=on  SaturateOnIntegerOverflow=on  OutDataTypeStr=Inherit: Same as first input
      mask Display: e = 0.06;c1 = [120 150 230]/255;c2 = ([120 150 230]+0)/383;c3 = ([120 150 230]+128)/383;patch([0 1 1 0],[0 0 1 1],c1);patch([0 1 1 1-e 1-e 0+e],[0 0 1 1-e 0+e 0+e],c2);patch([0 0 1 1-e 0+e 0+e],[0 1 1 1-e 1-e 0+e],c3);plot([0 1 1 0 0],[0 0 1 1 0]);disp('+');
  tansig : neural/Transfer Functions/tansig
  "a{1}" : Outport  InitialOutput=[0;0;0;0;0;0;0;0;0;0;0;0;0;0;0;0;0;0;0;0;0;0;0;0;0;0;0;0;0;0;0;0;0;0;0;0;0;0;0;0;0;0;0;0;0;0;0;0;0;0]
      mask Display: e = 0.06;c1 = [120 230 180]/255;c2 = ([120 230 180]+0)/(256+128);c3 = ([120 230 180]+128)/(256+128);patch([0 1 1 0],[0 0 1 1],c1);patch([0 1 1 1-e 1-e 0+e],[0 0 1 1-e 0+e 0+e],c2);patch([0 0 1 1-e 0+e 0+e],[0 1 1 1-e 1-e 0+e],c3);plot([0 1 1 0 0],[0 0 1 1 0]);
  wires:
  "p{1}"/1 -> Delays 1/1("p{1}")
  Delays 1/1("pd{1,1}") -> "IW{1,1}"/1("pd{1,1}")
  "IW{1,1}"/1("iz{1,1}") -> netsum/1
  "b{1}"/1 -> netsum/2
  netsum/1 -> tansig/1
  tansig/1 -> "a{1}"/1

== system e5_Quadrotor_stable_nn/NN/Layer 2 ==
  "a{1} " : Inport  PortDimensions=50
      mask Display: e = 0.06;c1 = [120 230 180]/255;c2 = ([120 230 180]+0)/(256+128);c3 = ([120 230 180]+128)/(256+128);patch([0 1 1 0],[0 0 1 1],c1);patch([0 1 1 1-e 1-e 0+e],[0 0 1 1-e 0+e 0+e],c2);patch([0 0 1 1-e 0+e 0+e],[0 1 1 1-e 1-e 0+e],c3);plot([0 1 1 0 0],[0 0 1 1 0]);
  Delays 1 : Subsystem
      mask Display: e = 0.06;c1 = [120 150 230]/255;c2 = ([120 150 230]+0)/383;c3 = ([120 150 230]+128)/383;patch([0 1 1 0],[0 0 1 1],c1);patch([0 1 1 1-e 1-e 0+e],[0 0 1 1-e 0+e 0+e],c2);patch([0 0 1 1-e 0+e 0+e],[0 1 1 1-e 1-e 0+e],c3);plot([0 1 1 0 0],[0 0 1 1 0]);disp('0');
  "LW{2,1}" : Subsystem
      mask Display: e = 0.06;c1 = [120 150 230]/255;c2 = ([120 150 230]+0)/383;c3 = ([120 150 230]+128)/383;patch([0 1 1 0],[0 0 1 1],c1);patch([0 1 1 1-e 1-e 0+e],[0 0 1 1-e 0+e 0+e],c2);patch([0 0 1 1-e 0+e 0+e],[0 1 1 1-e 1-e 0+e],c3);plot([0 1 1 0 0],[0 0 1 1 0]);disp('W');
  "b{2}" : Constant  Value=[1.28161781860947154854102336685173213481903076171875;1.24192246401782568909766268916428089141845703125]
      mask Display: e = 0.06;c1 = [120 150 230]/255;c2 = ([120 150 230]+0)/383;c3 = ([120 150 230]+128)/383;patch([0 1 1 0],[0 0 1 1],c1);patch([0 1 1 1-e 1-e 0+e],[0 0 1 1-e 0+e 0+e],c2);patch([0 0 1 1-e 0+e 0+e],[0 1 1 1-e 1-e 0+e],c3);plot([0 1 1 0 0],[0 0 1 1 0]);disp('b');
  netsum : Sum  Inputs=2  InputSameDT=on  SaturateOnIntegerOverflow=on  OutDataTypeStr=Inherit: Same as first input
      mask Display: e = 0.06;c1 = [120 150 230]/255;c2 = ([120 150 230]+0)/383;c3 = ([120 150 230]+128)/383;patch([0 1 1 0],[0 0 1 1],c1);patch([0 1 1 1-e 1-e 0+e],[0 0 1 1-e 0+e 0+e],c2);patch([0 0 1 1-e 0+e 0+e],[0 1 1 1-e 1-e 0+e],c3);plot([0 1 1 0 0],[0 0 1 1 0]);disp('+');
  tansig : neural/Transfer Functions/tansig
  "a{2}" : Outport  InitialOutput=[0;0]
      mask Display: e = 0.06;c1 = [120 230 180]/255;c2 = ([120 230 180]+0)/(256+128);c3 = ([120 230 180]+128)/(256+128);patch([0 1 1 0],[0 0 1 1],c1);patch([0 1 1 1-e 1-e 0+e],[0 0 1 1-e 0+e 0+e],c2);patch([0 0 1 1-e 0+e 0+e],[0 1 1 1-e 1-e 0+e],c3);plot([0 1 1 0 0],[0 0 1 1 0]);
  wires:
  "a{1} "/1 -> Delays 1/1("p{2}")
  Delays 1/1("pd{2,1}") -> "LW{2,1}"/1("ad{2,1}")
  "LW{2,1}"/1("lz{2,1}") -> netsum/1
  "b{2}"/1 -> netsum/2
  netsum/1 -> tansig/1
  tansig/1 -> "a{2}"/1

== system e5_Quadrotor_stable_nn/NN/Process Input 1 ==
  x : Inport  PortDimensions=15
      mask Display: e = 0.06;c1 = [120 230 180]/255;c2 = ([120 230 180]+0)/(256+128);c3 = ([120 230 180]+128)/(256+128);patch([0 1 1 0],[0 0 1 1],c1);patch([0 1 1 1-e 1-e 0+e],[0 0 1 1-e 0+e 0+e],c2);patch([0 0 1 1-e 0+e 0+e],[0 1 1 1-e 1-e 0+e],c3);plot([0 1 1 0 0],[0 0 1 1 0]);
  mapminmax : neural/Processing Functions/mapminmax  xmin=[3.43124452034659910282243799884e-05;0.000861098109347690978017386687071;0;0;0;0;-7.7003185079193718675164004317e-05;0;-0.0177130156218504447585004868415;-7.7003185079193718675164004317e-05;0;-0.0177130156218504447585004868415;-7.7003185079193718675164004317e-05;0;-0.0177130156218504447585004868415]  xmax=[0.290478472715819224791999886293;0.299196855135444139683897901705;0.290478472715819224791999886293;0.299196855135444139683897901705;0.290478472715819224791999886293;0.299196855135444139683897901705;8.37153844184080562487379473247e-05;0.341964637358954937074173585643;0.337708363299572378313229137348;8.37153844184080562487379473247e-05;0.341964637358954937074173585643;0.337708363299572378313229137348;8.37153844184080562487379473247e-05;0.341964637358954937074173585643;0.337708363299572378313229137348]  ymin=-1  ymax=1
  p : Outport  PortDimensions=15
      mask Display: e = 0.06;c1 = [120 230 180]/255;c2 = ([120 230 180]+0)/(256+128);c3 = ([120 230 180]+128)/(256+128);patch([0 1 1 0],[0 0 1 1],c1);patch([0 1 1 1-e 1-e 0+e],[0 0 1 1-e 0+e 0+e],c2);patch([0 0 1 1-e 0+e 0+e],[0 1 1 1-e 1-e 0+e],c3);plot([0 1 1 0 0],[0 0 1 1 0]);
  wires:
  x/1 -> mapminmax/1
  mapminmax/1 -> p/1

== system e5_Quadrotor_stable_nn/NN/Process Output 1 ==
  a : Inport  PortDimensions=2
      mask Display: e = 0.06;c1 = [120 230 180]/255;c2 = ([120 230 180]+0)/(256+128);c3 = ([120 230 180]+128)/(256+128);patch([0 1 1 0],[0 0 1 1],c1);patch([0 1 1 1-e 1-e 0+e],[0 0 1 1-e 0+e 0+e],c2);patch([0 0 1 1-e 0+e 0+e],[0 1 1 1-e 1-e 0+e],c3);plot([0 1 1 0 0],[0 0 1 1 0]);
  mapminmax_reverse : neural/Processing Functions/mapminmax_reverse  xmin=[-0.0290478472715819252547575501922;-0.0225523089146122887593826078501]  xmax=[0.0181937723673191685536121298128;0.0299196855135444167439473517334]  ymin=-1  ymax=1
  y : Outport  PortDimensions=2
      mask Display: e = 0.06;c1 = [120 230 180]/255;c2 = ([120 230 180]+0)/(256+128);c3 = ([120 230 180]+128)/(256+128);patch([0 1 1 0],[0 0 1 1],c1);patch([0 1 1 1-e 1-e 0+e],[0 0 1 1-e 0+e 0+e],c2);patch([0 0 1 1-e 0+e 0+e],[0 1 1 1-e 1-e 0+e],c3);plot([0 1 1 0 0],[0 0 1 1 0]);
  wires:
  a/1 -> mapminmax_reverse/1
  mapminmax_reverse/1 -> y/1

== system e5_Quadrotor_stable_nn/NN_online/Layer 1 ==
  "p{1}" : Inport  PortDimensions=20
      mask Display: e = 0.06;c1 = [120 230 180]/255;c2 = ([120 230 180]+0)/(256+128);c3 = ([120 230 180]+128)/(256+128);patch([0 1 1 0],[0 0 1 1],c1);patch([0 1 1 1-e 1-e 0+e],[0 0 1 1-e 0+e 0+e],c2);patch([0 0 1 1-e 0+e 0+e],[0 1 1 1-e 1-e 0+e],c3);plot([0 1 1 0 0],[0 0 1 1 0]);
  Delays 1 : Subsystem
      mask Display: e = 0.06;c1 = [120 150 230]/255;c2 = ([120 150 230]+0)/383;c3 = ([120 150 230]+128)/383;patch([0 1 1 0],[0 0 1 1],c1);patch([0 1 1 1-e 1-e 0+e],[0 0 1 1-e 0+e 0+e],c2);patch([0 0 1 1-e 0+e 0+e],[0 1 1 1-e 1-e 0+e],c3);plot([0 1 1 0 0],[0 0 1 1 0]);disp('0');
  "IW{1,1}" : Subsystem
      mask Display: e = 0.06;c1 = [120 150 230]/255;c2 = ([120 150 230]+0)/383;c3 = ([120 150 230]+128)/383;patch([0 1 1 0],[0 0 1 1],c1);patch([0 1 1 1-e 1-e 0+e],[0 0 1 1-e 0+e 0+e],c2);patch([0 0 1 1-e 0+e 0+e],[0 1 1 1-e 1-e 0+e],c3);plot([0 1 1 0 0],[0 0 1 1 0]);disp('W');
  "b{1}" : Constant  Value=[1.773843019974727486243182283942587673664093017578125;1.622878773289350373687511819298379123210906982421875;1.4561444625262309759960999144823290407657623291015625;1.381780857734258294300389025011099874973297119140625;-1.2744257887490910707839475435321219265460968017578125;1.2704629812613379424846016263472847640514373779296875;-0.94544009091574476855157627142034471035003662109375;-0.9337379344929856994639294498483650386333465576171875;-0.56109092582451458586234593894914723932743072509765625;-0.499047995113156950264254874127800576388835906982421875;-0.309368061599387844662345514734624885022640228271484375;0.3059387609359534021535864667384885251522064208984375;0.30987174868634070890038856305181980133056640625;-0.1240530062472051386901483738256501965224742889404296875;-0.2292650903033664200325603133023832924664020538330078125;0.1919116845205318389044890636796480976045131683349609375;-0.2367090426730429353341378373443149030208587646484375;0.632733666045173226422093648579902946949005126953125;-0.2539514671290665770442274151719175279140472412109375;0.273149558210549814329937134971260093152523040771484375;0.6098064760409156459530777283362112939357757568359375;-0.6655571849606707335311739370808936655521392822265625;-1.30952134522071705902135363430716097354888916015625;-1.124358574038685443241547545767389237880706787109375;-0.88408684534701631463349258410744369029998779296875;-1.070131743479656893924811811302788555622100830078125;-0.888301098263443833502606139518320560455322265625;1.60637678577253861789131406112574040889739990234375;-1.438485442130331914967200646060518920421600341796875;1.4975028639498424443132762462482787668704986572265625]
      mask Display: e = 0.06;c1 = [120 150 230]/255;c2 = ([120 150 230]+0)/383;c3 = ([120 150 230]+128)/383;patch([0 1 1 0],[0 0 1 1],c1);patch([0 1 1 1-e 1-e 0+e],[0 0 1 1-e 0+e 0+e],c2);patch([0 0 1 1-e 0+e 0+e],[0 1 1 1-e 1-e 0+e],c3);plot([0 1 1 0 0],[0 0 1 1 0]);disp('b');
  netsum : Sum  Inputs=2  InputSameDT=on  SaturateOnIntegerOverflow=on  OutDataTypeStr=Inherit: Same as first input
      mask Display: e = 0.06;c1 = [120 150 230]/255;c2 = ([120 150 230]+0)/383;c3 = ([120 150 230]+128)/383;patch([0 1 1 0],[0 0 1 1],c1);patch([0 1 1 1-e 1-e 0+e],[0 0 1 1-e 0+e 0+e],c2);patch([0 0 1 1-e 0+e 0+e],[0 1 1 1-e 1-e 0+e],c3);plot([0 1 1 0 0],[0 0 1 1 0]);disp('+');
  tansig : neural/Transfer Functions/tansig
  "a{1}" : Outport  InitialOutput=[0;0;0;0;0;0;0;0;0;0;0;0;0;0;0;0;0;0;0;0;0;0;0;0;0;0;0;0;0;0]
      mask Display: e = 0.06;c1 = [120 230 180]/255;c2 = ([120 230 180]+0)/(256+128);c3 = ([120 230 180]+128)/(256+128);patch([0 1 1 0],[0 0 1 1],c1);patch([0 1 1 1-e 1-e 0+e],[0 0 1 1-e 0+e 0+e],c2);patch([0 0 1 1-e 0+e 0+e],[0 1 1 1-e 1-e 0+e],c3);plot([0 1 1 0 0],[0 0 1 1 0]);
  wires:
  "p{1}"/1 -> Delays 1/1("p{1}")
  Delays 1/1("pd{1,1}") -> "IW{1,1}"/1("pd{1,1}")
  "IW{1,1}"/1("iz{1,1}") -> netsum/1
  "b{1}"/1 -> netsum/2
  netsum/1 -> tansig/1
  tansig/1 -> "a{1}"/1
